simulink model "CA1_model"  (R2023a)
settings: Solver=VariableStepAuto  StartTime=0.0  StopTime=50  RelTol=1e-3
values from neighbouring files (symbols this model uses):
  a1 = 0.22    [CA1.m]
  a2 = 6.1    [CA1.m]
  a_m = 3    [CA1.m]
  b0 = -0.5    [CA1.m]
  b1 = -1    [CA1.m]
  Gamma = 100*diag([1*ga,1*ga,1*ga,1*ga,1*ga])    [CA1.m]
  R_m = [1 a_m]    [CA1.m]
  T = [1 2*eta*wn wn^2]    [CA1.m]
  theta_bar_star = [K_star,-G1(3),-G1(2),-Fbar(4),-Fbar(3)]    [CA1.m]
settings Model: Creator=Administrator  LastModifiedBy=lwh
settings DebuggingCC: UnconnectedInputMsg=warning  UnconnectedOutputMsg=warning  UnconnectedLineMsg=warning
settings ModelReferenceCC: EnableRefExpFcnMdlSchedulingChecks=on
settings RTWCC: DLArmComputeVersion=19.05

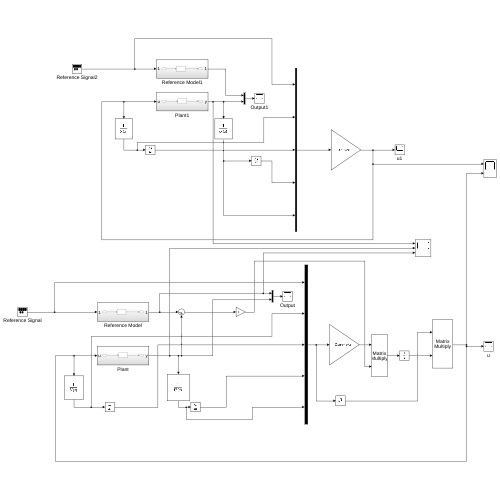
[thumbnail: Simulink's stored preview of the top-level diagram]
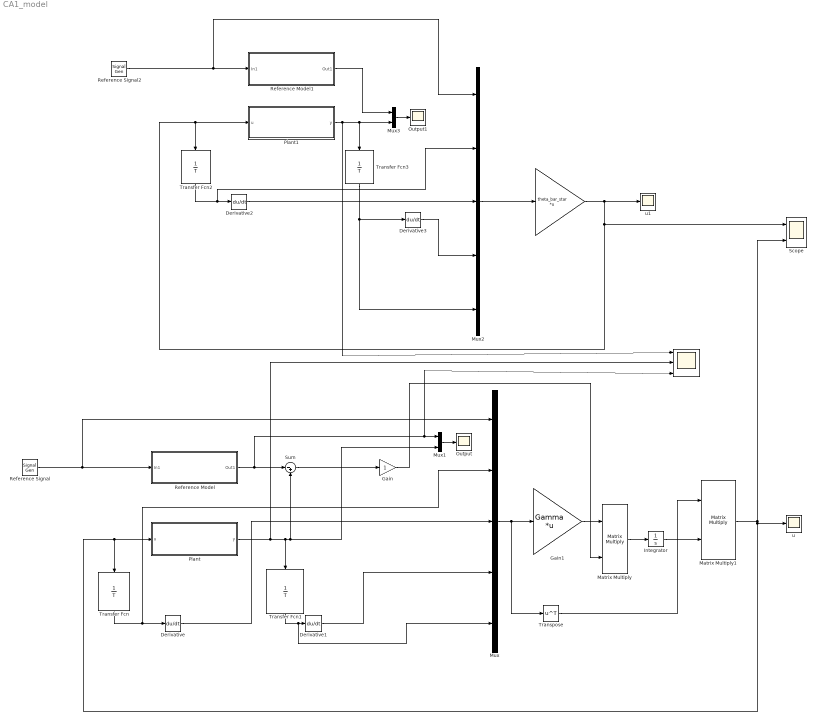
== system CA1_model ==
  " " : Scope  NumInputPorts=3
  "  " : Gain  Gain=theta_bar_star  Multiplication=Matrix(K*u) (u vector)
  Derivative{,1..3} (4 alike) : Derivative
  Gain : Gain
  Gain1 : Gain  Gain=Gamma  Multiplication=Matrix(K*u)
  Integrator : Integrator
  Matrix Multiply : Product  Multiplication=Matrix(*)
  Matrix Multiply1 : Product  Multiplication=Matrix(*)
  Mux : Mux  Inputs=5
  Mux1 : Mux  Inputs=2
  Mux2 : Mux  Inputs=5
  Mux3 : Mux  Inputs=2
  Output : Scope
  Output1 : Scope
  Plant : Subsystem
  Plant1 : Subsystem
  Reference Model : Subsystem
  Reference Model1 : Subsystem
  Reference Signal : SignalGenerator  WaveForm=square  Frequency=0.5
  Reference Signal2 : SignalGenerator  WaveForm=square  Frequency=0.5
  Scope : Scope  NumInputPorts=2
  Sum : Sum  Inputs=|-+
  Transfer Fcn{,1..3} (4 alike) : TransferFcn  Denominator=T
  Transpose : Math  Operator=transpose
  u : Scope
  u1 : Scope
  wires:
  Reference Model/1(Out1) -> Sum/1, " "/3, Mux1/1
  Plant/1(y) -> " "/2, Mux1/2, Sum/2, Transfer Fcn1/1
  Sum/1 -> Gain/1
  Reference Signal/1 -> Reference Model/1(In1), Mux/1
  Transfer Fcn/1 -> Mux/2, Derivative/1
  Derivative/1 -> Mux/3
  Transfer Fcn1/1 -> Mux/5, Derivative1/1
  Mux/1 -> Gain1/1, Transpose/1
  Matrix Multiply/1 -> Integrator/1
  Matrix Multiply1/1 -> Plant/1(u), Transfer Fcn/1, u/1, Scope/2
  Mux1/1 -> Output/1
  Transfer Fcn3/1 -> Mux2/5, Derivative3/1
  Mux2/1 -> "  "/1
  Derivative3/1 -> Mux2/4
  Derivative2/1 -> Mux2/3
  Reference Model1/1(Out1) -> Mux3/1
  Reference Signal2/1 -> Reference Model1/1(In1), Mux2/1
  Plant1/1(y) -> " "/1, Mux3/2, Transfer Fcn3/1
  Mux3/1 -> Output1/1
  Transfer Fcn2/1 -> Derivative2/1, Mux2/2
  "  "/1 -> u1/1, Plant1/1(u), Transfer Fcn2/1, Scope/1
  Derivative1/1 -> Mux/4
  Gain1/1 -> Matrix Multiply/1
  Gain/1 -> Matrix Multiply/2
  Integrator/1 -> Matrix Multiply1/2
  Transpose/1 -> Matrix Multiply1/1

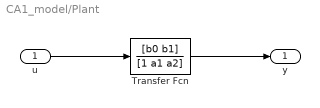
== system CA1_model/Plant ==
  u : Inport
  Transfer Fcn : TransferFcn  Numerator=[b0 b1]  Denominator=[1 a1 a2]
  y : Outport
  wires:
  u/1 -> Transfer Fcn/1
  Transfer Fcn/1 -> y/1

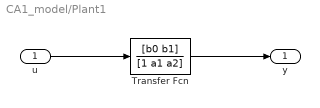
== system CA1_model/Plant1 ==
  u : Inport
  Transfer Fcn : TransferFcn  Numerator=[b0 b1]  Denominator=[1 a1 a2]
  y : Outport
  wires:
  u/1 -> Transfer Fcn/1
  Transfer Fcn/1 -> y/1

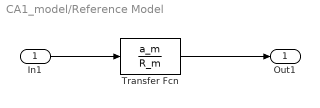
== system CA1_model/Reference Model ==
  In1 : Inport
  Transfer Fcn : TransferFcn  Numerator=a_m  Denominator=R_m
  Out1 : Outport
  wires:
  In1/1 -> Transfer Fcn/1
  Transfer Fcn/1 -> Out1/1

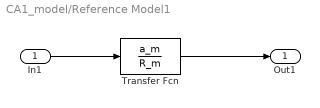
== system CA1_model/Reference Model1 ==
  In1 : Inport
  Transfer Fcn : TransferFcn  Numerator=a_m  Denominator=R_m
  Out1 : Outport
  wires:
  In1/1 -> Transfer Fcn/1
  Transfer Fcn/1 -> Out1/1
